simulink model "mux"  (R2018a)
settings: Solver=VariableStepAuto  StartTime=0.0  StopTime=10.0  RelTol=1e-3
settings Model: Creator=BEAR  LastModifiedBy=BEAR

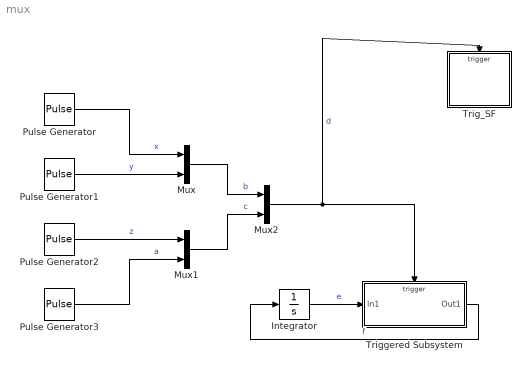
== system mux ==
  Integrator : Integrator  InitialCondition=-1
  Mux : Mux  Inputs=2
  Mux1 : Mux  Inputs=2
  Mux2 : Mux  Inputs=2
  Pulse Generator : DiscretePulseGenerator  PulseType=Time based  Period=10  PulseWidth=10
  Pulse Generator1 : DiscretePulseGenerator  PulseType=Time based  Period=10  PulseWidth=10  PhaseDelay=1
  Pulse Generator2 : DiscretePulseGenerator  PulseType=Time based  Period=10  PulseWidth=10  PhaseDelay=2
  Pulse Generator3 : DiscretePulseGenerator  PulseType=Time based  Period=10  PulseWidth=10  PhaseDelay=3
  Trig_SF : Stateflow chart  TreatAsAtomicUnit=on
  Triggered Subsystem : Subsystem  TreatAsAtomicUnit=on
  wires:
  Pulse Generator/1 -> Mux/1  "x"
  Pulse Generator1/1 -> Mux/2  "y"
  Pulse Generator2/1 -> Mux1/1  "z"
  Pulse Generator3/1 -> Mux1/2  "a"
  Mux/1 -> Mux2/1  "b"
  Mux1/1 -> Mux2/2  "c"
  Mux2/1 -> Trig_SF/Trigger, Triggered Subsystem/Trigger  "d"
  Integrator/1 -> Triggered Subsystem/1(In1)  "e"
  Triggered Subsystem/1(Out1) -> Integrator/1  "f"

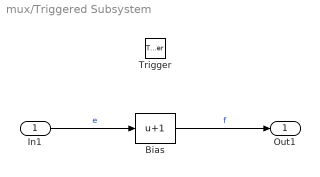
== system mux/Triggered Subsystem ==
  In1 : Inport
  Trigger : TriggerPort  VariantControl=Variant
  Bias : Bias  Bias=1
  Out1 : Outport
  wires:
  In1/1 -> Bias/1  "e"
  Bias/1 -> Out1/1  "f"

== stateflow chart mux/Trig_SF ==
  state A
  state B
    state B1
    state B2
    (default) -> B1
    B1 -> B2 : event2
    B2 -> B1 : event3
  (default) -> A
  A -> B : event
  B -> A : event1
  events: event input RISING_EDGE_EVENT; event1 input FALLING_EDGE_EVENT; event2 input EITHER_EDGE_EVENT; event3 input RISING_EDGE_EVENT
